simulink model "SbW_Model1"  (R2026a)
settings: Solver=ode45  StopTime=20  RelTol=1e-4
libraries: slpidlib x1
settings Model: Creator=walis  LastModifiedBy=Pai
settings DebuggingCC: InheritedTsInSrcMsg=none

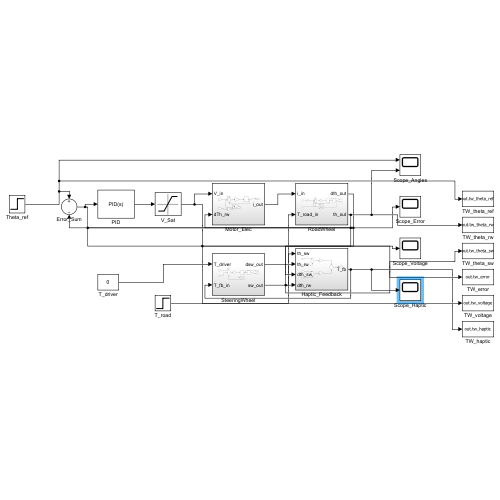
[thumbnail: Simulink's stored preview of the top-level diagram]
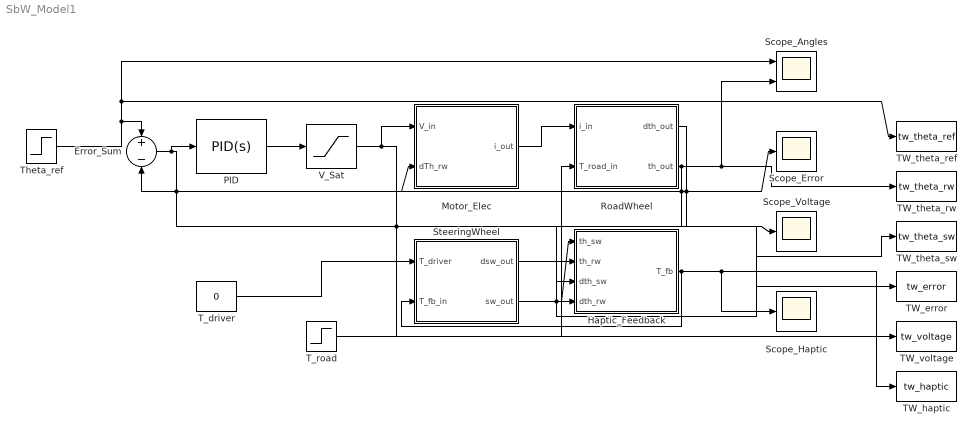
== system SbW_Model1 ==
  Error_Sum : Sum  Inputs=+-
  Haptic_Feedback : Subsystem
  Motor_Elec : Subsystem
  PID : slpidlib/PID Controller  Controller=PID  Form=Parallel  TimeDomain=Continuous-time  UseExternalTs=off  SampleTime=-1  IntegratorMethod=Forward Euler  FilterMethod=Forward Euler  ControllerParametersSource=internal  P=50  I=10  UseKiTs=off  D=2  UseExternalDerivativeSource=off  N=100  UseFilter=on  TunerSelectOption=Transfer Function Based (PID Tuner App)  InitialConditionSource=internal  InitialConditionForIntegrator=0  InitialConditionForFilter=0  DifferentiatorICPrevScaledInput=0  ExternalReset=none  TrackingMode=off  Kt=1  LimitOutput=off  SatLimitsSource=internal  UpperSaturationLimit=inf  LowerSaturationLimit=-inf  LinearizeAsGain=on  AntiWindupMode=none  Kb=1  LimitIntegrator=off  UpperIntegratorSaturationLimit=inf  LowerIntegratorSaturationLimit=-inf  POutMin=[]  POutMax=[]  IOutMin=[]  IOutMax=[]  DOutMin=[]  DOutMax=[]  NOutMin=[]  NOutMax=[]  SumOutMin=[]  SumOutMax=[]  SaturationOutMin=[]  SaturationOutMax=[]  PParamMin=[]  PParamMax=[]  IParamMin=[]  IParamMax=[]  DParamMin=[]  DParamMax=[]  NParamMin=[]  NParamMax=[]  KbParamMin=[]  KbParamMax=[]  KtParamMin=[]  KtParamMax=[]  KbOutMin=[]  KbOutMax=[]  KtOutMin=[]  KtOutMax=[]  IntegratorOutMin=[]  IntegratorOutMax=[]  FilterOutMin=[]  FilterOutMax=[]  SumI1OutMin=[]  SumI1OutMax=[]  SumI2OutMin=[]  SumI2OutMax=[]  SumI3OutMin=[]  SumI3OutMax=[]  SumI4OutMin=[]  SumI4OutMax=[]  SumDOutMin=[]  SumDOutMax=[]  DifferentiatorOutMin=[]  DifferentiatorOutMax=[]  FilterDiffOutCoefMin=[]  FilterDiffOutCoefMax=[]  ReciprocalOutMin=[]  ReciprocalOutMax=[]  SumDenOutMin=[]  SumDenOutMax=[]  SumNumOutMin=[]  SumNumOutMax=[]  DivideOutMin=[]  DivideOutMax=[]  UdiffTsProdOutMin=[]  UdiffTsProdOutMax=[]  NTsProdOutMin=[]  NTsProdOutMax=[]  UintegralTsProdOutMin=[]  UintegralTsProdOutMax=[]  UngainTsProdOutMin=[]  UngainTsProdOutMax=[]  ClampingZeroOutDataTypeStr=Inherit: Inherit via back propagation  ClampingZeroOutMin=[]  ClampingZeroOutMax=[]  FilterDenConstantOutDataTypeStr=Inherit: Inherit via back propagation  FilterDenConstantOutMin=[]  FilterDenConstantOutMax=[]  PCopyOutDataTypeStr=Inherit: Inherit via back propagation  PCopyOutMin=[]  PCopyOutMax=[]  NCopyOutDataTypeStr=Inherit: Inherit via back propagation  NCopyOutMin=[]  NCopyOutMax=[]  IntegratorContinuousStateAttributes=''  IntegratorStateMustResolveToSignalObject=off  IntegratorRTWStateStorageClass=Auto  FilterContinuousStateAttributes=''  FilterStateMustResolveToSignalObject=off  FilterRTWStateStorageClass=Auto  ParallelPVariant=InternalParameters  IdealPVariant=Disabled  IVariant=InternalParameters  DVariant=InternalParameters  IntegratorVariant=Continuous  SatVariant=Disabled  AWVariant=Passthrough  PCopyVariant=Disabled  TRVariant=Disabled  FdbkBlocksVariant=Forward  IdealPFdbkVariant=Disabled  SatFdbkVariant=Disabled  DerivativeFilterVariant=ContFilter  NVariant=InternalParameters  NCopyVariant=Disabled  FilterICVariant=InternalICsFilter  IntegratorICVariant=InternalICs  ExternalResetVariant=Disabled  TRSumVariant=Passthrough  SumFdbkVariant=Disabled  SumVariant=Sum_PID  TsampFilterVariant=InternalTs  TsampNgainVariant=Passthrough  TsampIntegralVariant=Disabled_SignalSpec  ExternalSaturationOutDataTypeStr=Inherit: Same as second input  DerivativeSourceVariant=ErrorSignal  PreIntVariant=InternalPreInt
  RoadWheel : Subsystem
  Scope_Angles : Scope  NumInputPorts=2
      settings: ActiveDisplayYMinimum=-0.062499999999999986  ActiveDisplayYMaximum=0.5625
  Scope_Error : Scope
      settings: ActiveDisplayYMinimum=-0.062499999999999986  ActiveDisplayYMaximum=0.5625
  Scope_Haptic : Scope
      settings: ActiveDisplayYMinimum=-1.3861578591203019  ActiveDisplayYMaximum=0.3978151046265026
  Scope_Voltage : Scope
      settings: ActiveDisplayYMinimum=-1.4999999999999996  ActiveDisplayYMaximum=13.5
  SteeringWheel : Subsystem
  TW_error : ToWorkspace  VariableName=tw_error  SampleTime=-1
  TW_haptic : ToWorkspace  VariableName=tw_haptic  SampleTime=-1
  TW_theta_ref : ToWorkspace  VariableName=tw_theta_ref  SampleTime=-1
  TW_theta_rw : ToWorkspace  VariableName=tw_theta_rw  SampleTime=-1
  TW_theta_sw : ToWorkspace  VariableName=tw_theta_sw  SampleTime=-1
  TW_voltage : ToWorkspace  VariableName=tw_voltage  SampleTime=-1
  T_driver : Constant  Value=0  SampleTime=0
  T_road : Step  Time=6  FinalValue=2  SampleTime=0
  Theta_ref : Step  FinalValue=0.5  SampleTime=0
  V_Sat : Saturate  UpperLimit=12  LowerLimit=-12
  wires:
  Theta_ref/1 -> Scope_Angles/1, TW_theta_ref/1, Error_Sum/1
  Error_Sum/1 -> Scope_Error/1, TW_error/1, PID/1
  PID/1 -> V_Sat/1
  V_Sat/1 -> Scope_Voltage/1, TW_voltage/1, Motor_Elec/1(V_in)
  Motor_Elec/1(i_out) -> RoadWheel/1(i_in)
  T_road/1 -> RoadWheel/2(T_road_in)
  RoadWheel/1(dth_out) -> Motor_Elec/2(dTh_rw), Haptic_Feedback/4(dth_rw)
  RoadWheel/2(th_out) -> Error_Sum/2, Haptic_Feedback/2(th_rw), Scope_Angles/2, TW_theta_rw/1
  T_driver/1 -> SteeringWheel/1(T_driver)
  SteeringWheel/2(sw_out) -> Haptic_Feedback/1(th_sw), TW_theta_sw/1
  SteeringWheel/1(dsw_out) -> Haptic_Feedback/3(dth_sw)
  Haptic_Feedback/1(T_fb) -> Scope_Haptic/1, TW_haptic/1, SteeringWheel/2(T_fb_in)

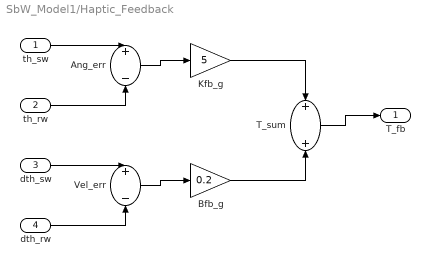
== system SbW_Model1/Haptic_Feedback ==
  th_sw : Inport
  th_rw : Inport  Port=2
  dth_sw : Inport  Port=3
  dth_rw : Inport  Port=4
  Ang_err : Sum  Inputs=+-
  Bfb_g : Gain  Gain=0.2
  Kfb_g : Gain  Gain=5
  T_sum : Sum
  Vel_err : Sum  Inputs=+-
  T_fb : Outport
  wires:
  th_sw/1 -> Ang_err/1
  th_rw/1 -> Ang_err/2
  dth_sw/1 -> Vel_err/1
  dth_rw/1 -> Vel_err/2
  Ang_err/1 -> Kfb_g/1
  Vel_err/1 -> Bfb_g/1
  Kfb_g/1 -> T_sum/1
  Bfb_g/1 -> T_sum/2
  T_sum/1 -> T_fb/1

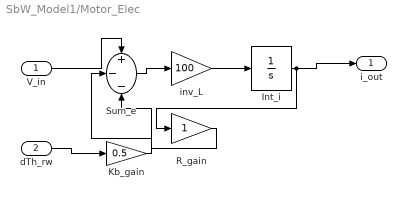
== system SbW_Model1/Motor_Elec ==
  V_in : Inport
  dTh_rw : Inport  Port=2
  Int_i : Integrator
  Kb_gain : Gain  Gain=0.5
  R_gain : Gain
  Sum_e : Sum  Inputs=+--
  inv_L : Gain  Gain=100
  i_out : Outport
  wires:
  V_in/1 -> Sum_e/1
  Sum_e/1 -> inv_L/1
  inv_L/1 -> Int_i/1
  Int_i/1 -> R_gain/1, i_out/1
  R_gain/1 -> Sum_e/2
  dTh_rw/1 -> Kb_gain/1
  Kb_gain/1 -> Sum_e/3

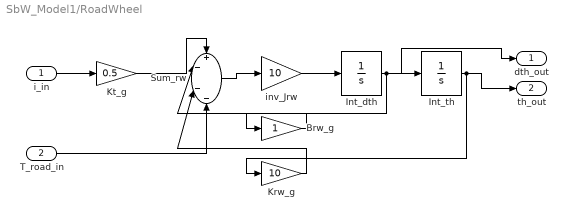
== system SbW_Model1/RoadWheel ==
  i_in : Inport
  T_road_in : Inport  Port=2
  Brw_g : Gain
  Int_dth : Integrator
  Int_th : Integrator
  Krw_g : Gain  Gain=10
  Kt_g : Gain  Gain=0.5
  Sum_rw : Sum  Inputs=+---
  inv_Jrw : Gain  Gain=10
  dth_out : Outport
  th_out : Outport  Port=2
  wires:
  i_in/1 -> Kt_g/1
  Kt_g/1 -> Sum_rw/1
  Sum_rw/1 -> inv_Jrw/1
  inv_Jrw/1 -> Int_dth/1
  Int_dth/1 -> Int_th/1, Brw_g/1, dth_out/1
  Brw_g/1 -> Sum_rw/2
  Int_th/1 -> Krw_g/1, th_out/1
  Krw_g/1 -> Sum_rw/3
  T_road_in/1 -> Sum_rw/4

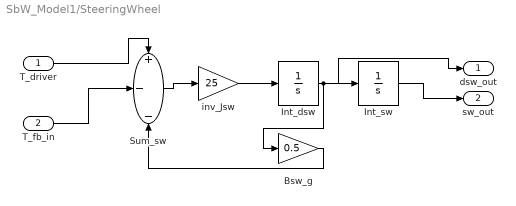
== system SbW_Model1/SteeringWheel ==
  T_driver : Inport
  T_fb_in : Inport  Port=2
  Bsw_g : Gain  Gain=0.5
  Int_dsw : Integrator
  Int_sw : Integrator
  Sum_sw : Sum  Inputs=+--
  inv_Jsw : Gain  Gain=25
  dsw_out : Outport
  sw_out : Outport  Port=2
  wires:
  T_driver/1 -> Sum_sw/1
  T_fb_in/1 -> Sum_sw/2
  Sum_sw/1 -> inv_Jsw/1
  inv_Jsw/1 -> Int_dsw/1
  Int_dsw/1 -> Int_sw/1, Bsw_g/1, dsw_out/1
  Bsw_g/1 -> Sum_sw/3
  Int_sw/1 -> sw_out/1
